simulink model "DashboardVCU"  (R2019b)
settings: Solver=VariableStepAuto  StartTime=0.0  StopTime=10.0  RelTol=1e-3

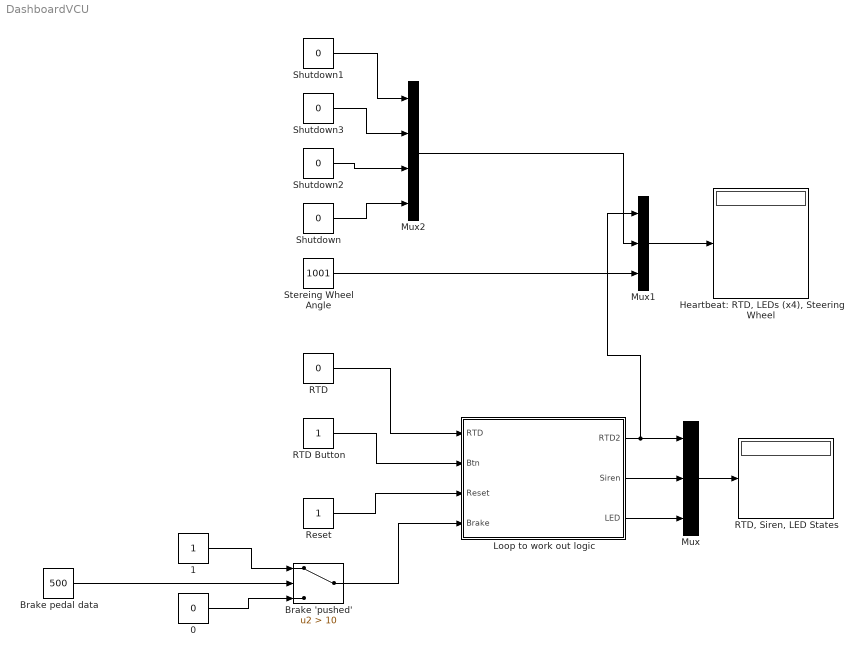
== system DashboardVCU ==
  0 : Constant  Value=0
  1 : Constant
  Brake 'pushed' : Switch  Criteria=u2 > Threshold  Threshold=10
  Brake pedal data : Constant  Value=500
  "Heartbeat: RTD, LEDs (x4), Steering Wheel" : Display
  Loop to work out logic : MATLAB Function  TreatAsAtomicUnit=on
  Mux : Mux  Inputs=3
  Mux1 : Mux  Inputs=3
  Mux2 : Mux
  RTD : Constant  Value=0
  RTD Button : Constant
  "RTD, Siren, LED States" : Display
  Reset : Constant
  Shutdown{,1..3} (4 alike) : Constant  Value=0
  Stereing Wheel Angle : Constant  Value=1001
  wires:
  RTD/1 -> Loop to work out logic/1(RTD)
  RTD Button/1 -> Loop to work out logic/2(Btn)
  Reset/1 -> Loop to work out logic/3(Reset)
  Loop to work out logic/3(LED) -> Mux/3
  Loop to work out logic/2(Siren) -> Mux/2
  Loop to work out logic/1(RTD2) -> Mux1/1, Mux/1
  Mux/1 -> "RTD, Siren, LED States"/1
  Brake pedal data/1 -> Brake 'pushed'/2
  1/1 -> Brake 'pushed'/1
  0/1 -> Brake 'pushed'/3
  Brake 'pushed'/1 -> Loop to work out logic/4(Brake)
  Mux1/1 -> "Heartbeat: RTD, LEDs (x4), Steering Wheel"/1
  Stereing Wheel Angle/1 -> Mux1/3
  Shutdown1/1 -> Mux2/1
  Shutdown/1 -> Mux2/4
  Mux2/1 -> Mux1/2
  Shutdown3/1 -> Mux2/2
  Shutdown2/1 -> Mux2/3

== matlab function DashboardVCU/Loop to work out logic ==
  data: RTD input; RTD2 output; Btn input; Reset input; Brake input; Siren output; LED output
function [RTD2,Siren,LED] = DashboardLogic(RTD, Btn, Reset, Brake)

if (RTD == 1)
    if (Btn == 1)
        RTD2 = 1;
        Siren = 1;
        LED = 1;
    else % Btn == 0
        RTD2 = 1;
        Siren = 0;
        LED = 1;
    end
else % RTD == 0
    if (Reset == 1)
        if (Brake == 1)
            if (Btn == 1)
                RTD2 = 1;
                Siren = 0;
                LED = 1; % In this scenario LED would flash
            else % Btn == 0
                RTD2 = 0;
                Siren = 0;
                LED = 1;
            end
        else % Brake == 0
            RTD2 = 0;
            Siren = 0;
            LED = 0;
        end
    else % Reset == 0
        RTD2 = 0;
        Siren = 0;
        LED = 0;
    end
end


end
